simulink model "calibrazione_acc_mag"  (Simulink 7.7)
settings: Solver=ode4  StartTime=0.0  StopTime=10.0  RelTol=1e-3
undefined symbols (not defined in the file): aerosimlib, Earth, WGS, WMM
libraries: aerolibgravity2 x1
settings Model: Creator=Fede  LastModifiedBy=Fede
settings OptimizationCC: OptimizeModelRefInitCode=on  LifeSpan=1
settings RTWCC: SystemTargetFile=ert.tlc  TemplateMakefile=ert_default_tmf  Description=Embedded Coder  ProcessScript=ert_make_rtw_hook
settings CodeAppCC: IgnoreCustomStorageClasses=off
settings ERTTargetCC: FunctionExecutionProfile=off  MultiwordLength=2048  GenerateSampleERTMain=on  ERTCustomFileTemplate=example_file_process.tlc  ConvertIfToSwitch=off

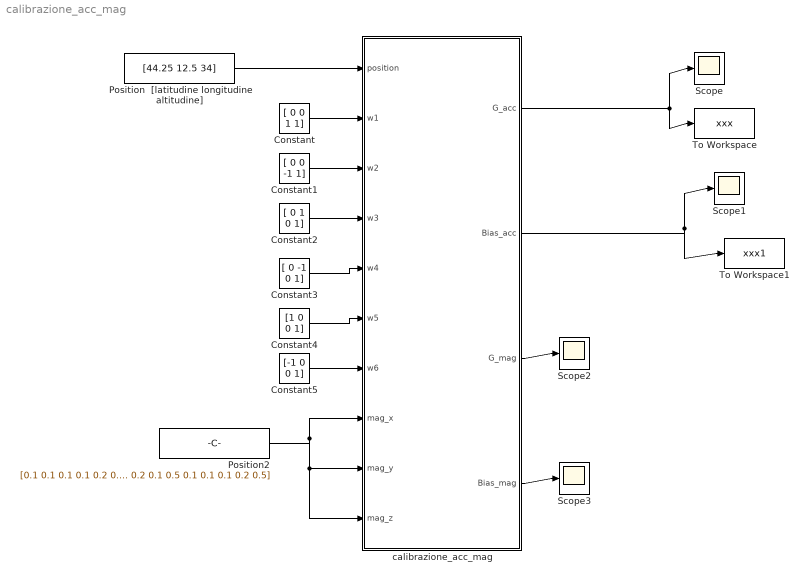
== system calibrazione_acc_mag ==
  Constant : Constant  Value=[ 0 0 1 1]
  Constant1 : Constant  Value=[ 0 0 -1 1]
  Constant2 : Constant  Value=[ 0 1 0 1]
  Constant3 : Constant  Value=[ 0 -1 0 1]
  Constant4 : Constant  Value=[1 0 0 1]
  Constant5 : Constant  Value=[-1 0 0 1]
  Position  [latitudine longitudine altitudine] : Constant  Value=[44.25 12.5 34]
  Position2 : Constant  Value=[0.1 0.1 0.1 0.1 0.2 0.1 0.5 0.1 0.1 0.1 0.2 0.5 0.1 0.1 0.1 0.1 0.2 0.1 0.5 0.1 0.1 0.1 0.2 0.5 0.1 0.1 0.1 0.1 0.2 0.1 0.5 0.1 0.1 0.1 0.2 0.5 0.1 0.1 0.1 0.1 0.2 0.1 0.5 0.1 0.1 0.1 0.2 0.5 0.1 0.1 0.1 0.1 0.2 0.1 0.5 0.1 0.1 0.1 0.2 0.5 0.1 0.1 0.1 0.1 0.2 0.1 0.5 0.1 0.1 0.1 0.2 0.5 0.1 0.1 0.1 0.1 0.2 0.1 0.5 0.1 0.1 0.1 0.2 0.5 0.1 0.1 0.1 0.1 0.2 0.1 0.5 0.1 0.1 0.1 0.2 0.5 0.1 0.1 0.1 0.1 0.2 0.1 0.5 0.1 0.1 0.1 0.2 0.5 0.1 0.1 0.1 0.1 0.2 0.1 0.5 0.1 0.1 0.1 0.2 0.5 0.1 0.1 0.1 0.1 0.2 0.1 0.5 0.1 0.1 0.1 0.2 0.5 0.1 0.1 0.1 0.1 0.2 0.1 0.5 0.1 0.1 0.1 0.2 0.5 0.1 0.1 0.1 0.1 0.2 0.1 0.5 0.1 0.1 0.1 0.2 0.5 0.1 0.1 0.1 0.1 0.2 0.1 0.5 0.1 0.1 0.1 0.2 0.5]
  Scope{,1..3} (4 alike) : Scope
      Scope2 settings: SaveName=ScopeData2
      Scope3 settings: SaveName=ScopeData3
  To Workspace : ToWorkspace  VariableName=xxx  SampleTime=-1  SaveFormat=Array
  To Workspace1 : ToWorkspace  VariableName=xxx1  SampleTime=-1  SaveFormat=Array
  calibrazione_acc_mag : Subsystem
  wires:
  Constant/1 -> calibrazione_acc_mag/2(w1)
  Constant1/1 -> calibrazione_acc_mag/3(w2)
  Constant2/1 -> calibrazione_acc_mag/4(w3)
  Constant3/1 -> calibrazione_acc_mag/5(w4)
  Constant4/1 -> calibrazione_acc_mag/6(w5)
  Constant5/1 -> calibrazione_acc_mag/7(w6)
  Position  [latitudine longitudine altitudine]/1 -> calibrazione_acc_mag/1(position)
  calibrazione_acc_mag/2(Bias_acc) -> Scope1/1, To Workspace1/1
  calibrazione_acc_mag/1(G_acc) -> To Workspace/1, Scope/1
  Position2/1 -> calibrazione_acc_mag/8(mag_x), calibrazione_acc_mag/9(mag_y), calibrazione_acc_mag/10(mag_z)
  calibrazione_acc_mag/3(G_mag) -> Scope2/1
  calibrazione_acc_mag/4(Bias_mag) -> Scope3/1

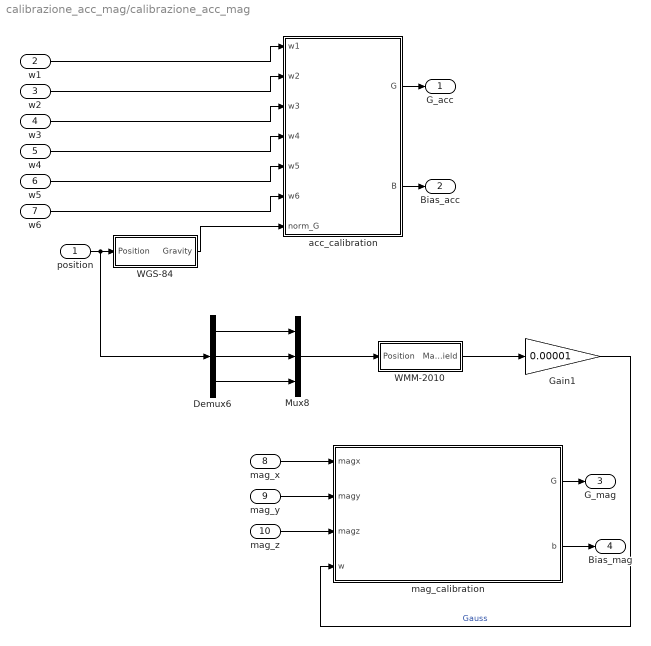
== system calibrazione_acc_mag/calibrazione_acc_mag ==
  position : Inport
  w1 : Inport  Port=2
  w2 : Inport  Port=3
  w3 : Inport  Port=4
  w4 : Inport  Port=5
  w5 : Inport  Port=6
  w6 : Inport  Port=7
  mag_x : Inport  Port=8
  mag_y : Inport  Port=9
  mag_z : Inport  Port=10
  Demux6 : Demux  Outputs=3
  Gain1 : Gain  Gain=0.00001
  Mux8 : Mux  Inputs=3
  WGS-84 : Subsystem  AncestorBlock=aerosimlib/Earth/WGS-84
      mask Type: WGS-84 Earth model
      mask Description: The WGS-84 Earth model provides local Earth radii and gravity as a function of position.
      mask Help:
      | The block provides a WGS-84 geoid model of the Earth.
      | <P><B>Inputs:</B>
      | <LI>Position = current aircraft location [Latitude Longitude Altitude], in [rad rad m]</LI>
      | </P>
      | <P><B>Output:</B>
      | <LI>Rmeridian = the Earth meridian radius, in m</LI>
      | <LI>Rnormal = the Earth normal radius, in m</LI>
      | <LI>Re = the Earth equivalent radius, in m</LI>
      | <LI>Gravity = the normal gravity, in m/s^2</LI>
      | </P>
  WMM-2010 : Subsystem  AncestorBlock=aerosimlib/Earth/WMM-2000  mask(WMM-2000){wmmfile='C:\\Programmmi\\AeroSim\\wmm.cof', simdate=[26 05 2011]}
      mask prompts: wmmfile "WMM coefficient file:"; simdate "Simulation date [Day Month Year]:"
      mask help: The World Magnetic Model returns the Earth magnetic field components in body axes at current aircraft location.
      mask Help:
      | The block provides the magnetic field components at current aircraft location.
      | <P><B>Inputs:</B>
      | <LI>Position = the 3x1 vector of aircraft location [Latitude Longitude Altitude] in [rad rad m]</LI>
      | <LI>DCM = the frame transformation matrix from navigation to body frame</LI>
      | </P>
      | <P><B>Output:</B>
      | <LI>MagField = the 3x1 vector of magnetic field components in body axes</LI>
      | </P>
      | <P><B>Parameters:</B>
      | <LI>WMM coefficient file = the path to the WMM coefficient file, as a 'string'</LI>
      | <LI>Simulation date = the 1x3 vector of current date [Day Month Year]</LI>
      | </P>
  acc_calibration : Stateflow chart  TreatAsAtomicUnit=on
  mag_calibration : Stateflow chart  TreatAsAtomicUnit=on
  G_acc : Outport
  Bias_acc : Outport  Port=2
  G_mag : Outport  Port=3
  Bias_mag : Outport  Port=4
  wires:
  position/1 -> WGS-84/1(Position), Demux6/1
  w1/1 -> acc_calibration/1(w1)
  w2/1 -> acc_calibration/2(w2)
  acc_calibration/1(G) -> G_acc/1
  w3/1 -> acc_calibration/3(w3)
  w4/1 -> acc_calibration/4(w4)
  w5/1 -> acc_calibration/5(w5)
  acc_calibration/2(B) -> Bias_acc/1
  w6/1 -> acc_calibration/6(w6)
  WGS-84/1(Gravity) -> acc_calibration/7(norm_G)
  Demux6/2 -> Mux8/2
  Demux6/1 -> Mux8/1
  Demux6/3 -> Mux8/3
  WMM-2010/1(MagField) -> Gain1/1
  Mux8/1 -> WMM-2010/1(Position)
  mag_x/1 -> mag_calibration/1(magx)
  mag_y/1 -> mag_calibration/2(magy)
  mag_calibration/1(G) -> G_mag/1
  mag_z/1 -> mag_calibration/3(magz)
  mag_calibration/2(b) -> Bias_mag/1
  Gain1/1 -> mag_calibration/4(w)  "Gauss"

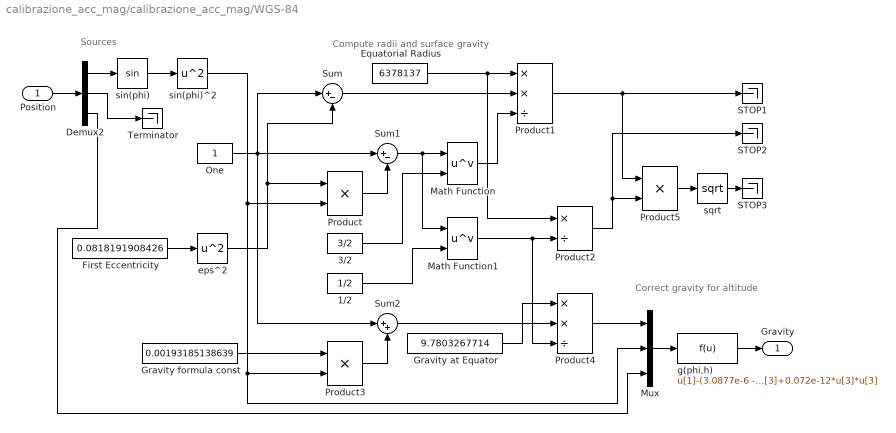
== system calibrazione_acc_mag/calibrazione_acc_mag/WGS-84 ==
  note: Correct gravity for altitude
  note: Compute radii and surface gravity
  note: Sources
  Position : Inport
  1/2 : Constant  Value=1/2
  3/2 : Constant  Value=3/2
  Demux2 : Demux  Outputs=3
  Equatorial Radius : Constant  Value=6378137
  First Eccentricity : Constant  Value=0.0818191908426
  Gravity at Equator : Constant  Value=9.7803267714
  Gravity formula const : Constant  Value=0.00193185138639
  Math Function : Math  Operator=pow  SaturateOnIntegerOverflow=on
  Math Function1 : Math  Operator=pow  SaturateOnIntegerOverflow=on
  Mux : Mux  Inputs=3
  One : Constant
  Product : Product  SaturateOnIntegerOverflow=on  InputSameDT=on  OutDataTypeStr=Inherit: Same as first input
  Product1 : Product  Inputs=**/  SaturateOnIntegerOverflow=on  InputSameDT=on  OutDataTypeStr=Inherit: Same as first input
  Product2 : Product  Inputs=*/  SaturateOnIntegerOverflow=on  InputSameDT=on  OutDataTypeStr=Inherit: Same as first input
  Product3 : Product  SaturateOnIntegerOverflow=on  InputSameDT=on  OutDataTypeStr=Inherit: Same as first input
  Product4 : Product  Inputs=**/  SaturateOnIntegerOverflow=on  InputSameDT=on  OutDataTypeStr=Inherit: Same as first input
  Product5 : Product  SaturateOnIntegerOverflow=on  InputSameDT=on  OutDataTypeStr=Inherit: Same as first input
  STOP1 : Terminator
  STOP2 : Terminator
  STOP3 : Terminator
  Sum : Sum  Inputs=|+-  SaturateOnIntegerOverflow=on  InputSameDT=on  OutDataTypeStr=Inherit: Same as first input
  Sum1 : Sum  Inputs=|+-  SaturateOnIntegerOverflow=on  InputSameDT=on  OutDataTypeStr=Inherit: Same as first input
  Sum2 : Sum  Inputs=|++  SaturateOnIntegerOverflow=on  InputSameDT=on  OutDataTypeStr=Inherit: Same as first input
  Terminator : Terminator
  eps^2 : Math  Operator=square  SaturateOnIntegerOverflow=on
  g(phi,h) : Fcn  Expr=u[1]-(3.0877e-6 - 0.0044e-6*u[2])*u[3]+0.072e-12*u[3]*u[3]
  sin(phi) : Trigonometry
  sin(phi)^2 : Math  Operator=square  SaturateOnIntegerOverflow=on
  sqrt : Math  Operator=sqrt  SaturateOnIntegerOverflow=on
  Gravity : Outport
  wires:
  Demux2/3 -> Mux/3
  g(phi,h)/1 -> Gravity/1
  Mux/1 -> g(phi,h)/1
  Demux2/2 -> Terminator/1
  Demux2/1 -> sin(phi)/1
  Position/1 -> Demux2/1
  Product4/1 -> Mux/1
  Sum2/1 -> Product4/2
  Gravity at Equator/1 -> Product4/1
  Product3/1 -> Sum2/2
  Gravity formula const/1 -> Product3/1
  Product2/1 -> Product5/2, STOP2/1
  Product1/1 -> Product5/1, STOP1/1
  Math Function1/1 -> Product4/3, Product2/2
  Math Function/1 -> Product1/3
  Sum/1 -> Product1/2
  Equatorial Radius/1 -> Product2/1, Product1/1
  1/2/1 -> Math Function1/2
  3/2/1 -> Math Function/2
  Sum1/1 -> Math Function1/1, Math Function/1
  Product/1 -> Sum1/2
  One/1 -> Sum/1, Sum2/1, Sum1/1
  sin(phi)^2/1 -> Mux/2, Product3/2, Product/2
  sin(phi)/1 -> sin(phi)^2/1
  eps^2/1 -> Product/1, Sum/2
  First Eccentricity/1 -> eps^2/1
  Product5/1 -> sqrt/1
  sqrt/1 -> STOP3/1

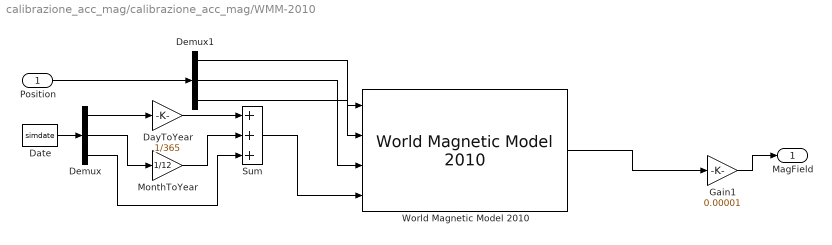
== system calibrazione_acc_mag/calibrazione_acc_mag/WMM-2010 ==
  Position : Inport  OutDataTypeStr=double  PortDimensions=[3 1]
  Date : Constant  Value=simdate
  DayToYear : Gain  Gain=1/365  SaturateOnIntegerOverflow=on  OutDataTypeStr=Inherit: Same as input  ParamDataTypeStr=Inherit: Same as input
  Demux : Demux  Outputs=3
  Demux1 : Demux  Outputs=3
  Gain1 : Gain  Gain=0.00001
  MonthToYear : Gain  Gain=1/12  SaturateOnIntegerOverflow=on  OutDataTypeStr=Inherit: Same as input  ParamDataTypeStr=Inherit: Same as input
  Sum : Sum  Inputs=+++  SaturateOnIntegerOverflow=on  InputSameDT=on  OutDataTypeStr=Inherit: Same as first input
  World Magnetic Model 2010 : aerolibgravity2/World Magnetic Model 2010  SystemSampleTime=-1  units=Metric (MKS)  time_in=on  month=January  day=1  year=2010  action=Error  h_out=off  dec_out=off  inc_out=off  ti_out=off
  MagField : Outport
  wires:
  Sum/1 -> World Magnetic Model 2010/4
  MonthToYear/1 -> Sum/2
  Demux/3 -> Sum/3
  Demux/2 -> MonthToYear/1
  DayToYear/1 -> Sum/1
  Demux/1 -> DayToYear/1
  Date/1 -> Demux/1
  Position/1 -> Demux1/1
  Demux1/1 -> World Magnetic Model 2010/2
  Demux1/2 -> World Magnetic Model 2010/3
  Demux1/3 -> World Magnetic Model 2010/1
  Gain1/1 -> MagField/1
  World Magnetic Model 2010/1 -> Gain1/1

== matlab function calibrazione_acc_mag/mag_calibration ==
  data: magx input double; G output double; magy input double; magz input double; w input double; b output double
function [G,b] = fcn(magx, magy,magz,w)
%#codegen
n=40;
%H=[];
H=zeros(n,10);
Hb=zeros(n,3);
B=zeros(n,3);
G=zeros(3,3);
%f=[0:1000:1];
%j=[0:1000:1];
%k=[0:1000:1];
%B=[];
%G=[];
%Hb=[];
h=w(1,:);
hx=magx;
hy=magy;
hz=magz;
for i=1:1:10    %per far si che H abbia almeno 10 elemnti così m>n
    H(i,1)=hx(i)^2;
    H(i,2)=2*hx(i)*hy(i);
    H(i,3)=2*hx(i)*hz(i);
    H(i,4)=hy(i)^2;
    H(i,5)=2*hy(i)*hz(i);
    H(i,6)=hz(i)^2;
    H(i,7)=hx(i);
    H(i,8)=hy(i);
    H(i,9)=hz(i);
    H(i,10)=1;
    Hb(i,1)=hx(i);
    Hb(i,2)=hy(i);
    Hb(i,3)=hz(i);
end
%for i=11:1:length(magx)-1 %ora inizia l'algoritmo
for i=11:1:n -1 %ora inizia l'algoritmo

    H(i,1)=hx(i)^2;
    H(i,2)=2*hx(i)*hy(i);
    H(i,3)=2*hx(i)*hz(i);
    H(i,4)=hy(i)^2;
    H(i,5)=2*hy(i)*hz(i);
    H(i,6)=hz(i)^2;
    H(i,7)=hx(i);
    H(i,8)=hy(i);
    H(i,9)=hz(i);
    H(i,10)=1;
    HH=H'*H; % uso la notazione dell'articolo e creo HH
    [K,P,L]=svd(HH); %HH è una matrice quadrata da cui k è uguale a L
    gsi_norm=K(:,10); % mi fido dell'articolo e prendo la decima colonna che in effetti è relativa al 10° valore singolare che è il + piccolo
    g1=gsi_norm(1);
    g2=gsi_norm(2);
    g3=gsi_norm(3);
    g4=gsi_norm(4);
    g5=gsi_norm(5);
    g6=gsi_norm(6);
    g7=gsi_norm(7);
    g8=gsi_norm(8);
    g9=gsi_norm(9);
    g10=gsi_norm(10);
    gamma=[g1 g2 g3;g2 g4 g5;g3 g5 g6];
    b=-0.5*inv(gamma)*[g7;g8;g9];
    bx=b(1);
    by=b(2);
    bz=b(3);
    B(i,1)=bx; %creo B per notare una convergenza
    B(i,2)=by;
    B(i,3)=bz;
    gsi_modulo=h*h'*(g1*bx^2+2*g2*bx*by+2*g3*bx*bz+g4*by^2+2*g5*by*bz+2*g6*bz^2-g10)^-1; % credo di poter elevare alla -1 tanto è uno scalare
    gsi=gsi_norm*gsi_modulo;
    g1=gsi(1);
    g2=gsi(2);
    g3=gsi(3);
    g4=gsi(4);
    g5=gsi(5);
    g6=gsi(6);
    g7=gsi(7);
    g8=gsi(8);
    g9=gsi(9);
    g10=gsi(10);
    gamma=[g1 g2 g3;g2 g4 g5;g3 g5 g6];
    [U,A,V]=svd(gamma); %per come è costruita gamma è quadrata e simmetrica da cui U è uguale a V
    G=V*sqrt(A)*V';
    b=[bx;by;bz];
    hm=[hx(i);hy(i);hz(i)];
    hb=G*(hm-b);
    Hb(i,1)=hb(1);
    Hb(i,2)=hb(2);
    Hb(i,3)=hb(3);
    %f(i)=norm(hm); %norma del vettore misurato
    %j(i)=norm(hb); %norma del vettore calibrato
    %k(i)=norm(h);  %norma del vettore reale
   
end

== matlab function calibrazione_acc_mag/acc_calibration ==
  data: w1 input double; G output double; w2 input double; w3 input double; w4 input double; w5 input double; w6 input double; B output double; norm_G input double
function [G, B] = fcn(w1,w2,w3,w4,w5,w6,norm_G)
%#codegen
Y=[ 0 ,0 ,norm_G;
    0 ,0, -norm_G;
    0 ,norm_G ,0;
    0, -norm_G, 0;
    norm_G ,0 ,0;
    -norm_G ,0, 0];

W=[w1,w2,w3,w4,w5,w6]';
X=((inv(W'*W))*W')*Y;
G=[X(1,1),X(1,2),X(1,3);
    X(2,1),X(2,2),X(2,3);
    X(3,1),X(3,2),X(3,3)];
B=[X(4,1),X(4,2),X(4,3)];
%X=(inv(W'*W))*W'*Y;
